simulink model "q2"  (R2020b)
settings: Solver=VariableStepAuto  StartTime=0.0  StopTime=10.0  RelTol=1e-3
values from neighbouring files (symbols this model uses):
  be = 2.0    [clutchpedal_data.sldd]
  bv = 1.0    [clutchpedal_data.sldd]
  Ie = 1.0    [clutchpedal_data.sldd]
  Iv = 5.0    [clutchpedal_data.sldd]
  muk = 1.0    [clutchpedal_data.sldd]
  mus = 1.5    [clutchpedal_data.sldd]
  R = 1.0    [clutchpedal_data.sldd]
settings Model: DataDictionary=clutchpedal_data.sldd  OrderedModelArguments=off  Creator=Ravi  LastModifiedBy=Ravi

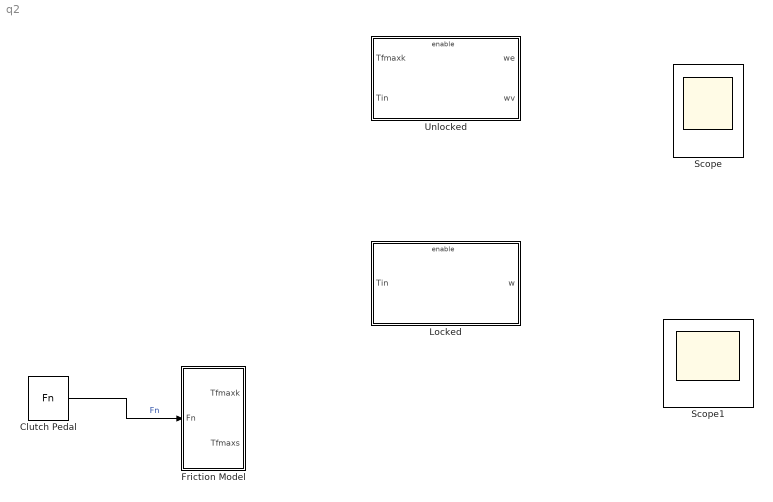
== system q2 ==
  Clutch Pedal : FromWorkspace  VariableName=Fn
  Friction Model : Subsystem
  Locked : Subsystem
  Scope : Scope  NumInputPorts=4
  Scope1 : Scope  NumInputPorts=4
  Unlocked : Subsystem
  wires:
  Clutch Pedal/1 -> Friction Model/1(Fn)  "Fn"

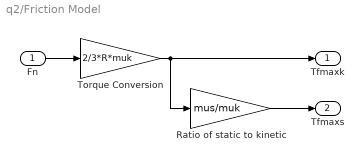
== system q2/Friction Model ==
  Fn : Inport
  Ratio of static to kinetic : Gain  Gain=mus/muk  SaturateOnIntegerOverflow=on  OutDataTypeStr=Inherit: Same as input  ParamDataTypeStr=Inherit: Same as input
  Torque Conversion : Gain  Gain=2/3*R*muk  SaturateOnIntegerOverflow=on  OutDataTypeStr=Inherit: Same as input  ParamDataTypeStr=Inherit: Same as input
  Tfmaxk : Outport  InitialOutput=0  VectorParamsAs1DForOutWhenUnconnected=off
  Tfmaxs : Outport  Port=2  InitialOutput=0  VectorParamsAs1DForOutWhenUnconnected=off
  wires:
  Ratio of static to kinetic/1 -> Tfmaxs/1
  Torque Conversion/1 -> Tfmaxk/1, Ratio of static to kinetic/1
  Fn/1 -> Torque Conversion/1

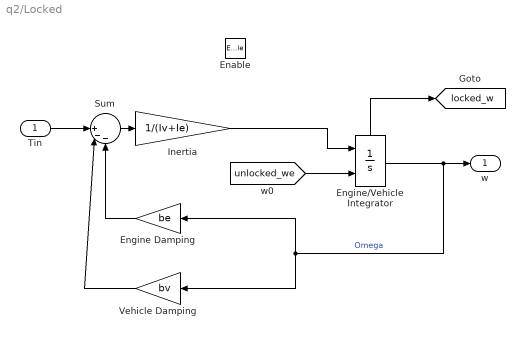
== system q2/Locked ==
  Tin : Inport
  Enable : EnablePort  StatesWhenEnabling=reset
  Engine Damping : Gain  Gain=be  SaturateOnIntegerOverflow=on  OutDataTypeStr=Inherit: Same as input  ParamDataTypeStr=Inherit: Same as input
  Engine/Vehicle Integrator : Integrator  InitialConditionSource=external  ShowStatePort=on
  Inertia : Gain  Gain=1/(Iv+Ie)  SaturateOnIntegerOverflow=on  OutDataTypeStr=Inherit: Same as input  ParamDataTypeStr=Inherit: Same as input
  Sum : Sum  Inputs=||+--  InputSameDT=on  SaturateOnIntegerOverflow=on  OutDataTypeStr=Inherit: Same as first input
  Vehicle Damping : Gain  Gain=bv  SaturateOnIntegerOverflow=on  OutDataTypeStr=Inherit: Same as input  ParamDataTypeStr=Inherit: Same as input
  w : Outport  InitialOutput=0  VectorParamsAs1DForOutWhenUnconnected=off
  tag scope: locked_w=global
  wires:
  Vehicle Damping/1 -> Sum/2
  Inertia/1 -> Engine/Vehicle Integrator/1
  Engine Damping/1 -> Sum/3
  Engine/Vehicle Integrator/1 -> Vehicle Damping/1, Engine Damping/1, w/1  "Omega"
  Tin/1 -> Sum/1
  Sum/1 -> Inertia/1
  Engine/Vehicle Integrator/State -> [locked_w]
  [unlocked_we] -> Engine/Vehicle Integrator/2

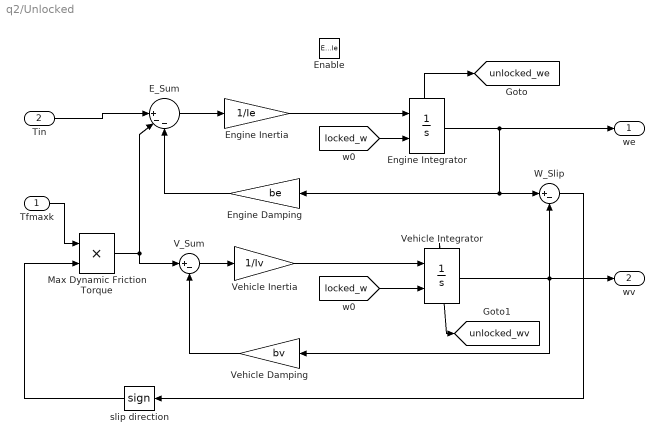
== system q2/Unlocked ==
  Tfmaxk : Inport
  Tin : Inport  Port=2
  Enable : EnablePort  StatesWhenEnabling=reset
  E_Sum : Sum  Inputs=||+--  InputSameDT=on  SaturateOnIntegerOverflow=on  OutDataTypeStr=Inherit: Same as first input
  Engine Damping : Gain  Gain=be  SaturateOnIntegerOverflow=on  OutDataTypeStr=Inherit: Same as input  ParamDataTypeStr=Inherit: Same as input
  Engine Inertia : Gain  Gain=1/Ie  SaturateOnIntegerOverflow=on  OutDataTypeStr=Inherit: Same as input  ParamDataTypeStr=Inherit: Same as input
  Engine Integrator : Integrator  InitialConditionSource=external  ShowStatePort=on
  Max Dynamic Friction Torque : Product  InputSameDT=on  RndMeth=Zero  SaturateOnIntegerOverflow=on  OutDataTypeStr=Inherit: Same as first input
  V_Sum : Sum  Inputs=|+-  InputSameDT=on  SaturateOnIntegerOverflow=on  OutDataTypeStr=Inherit: Same as first input
  Vehicle Integrator : Integrator  InitialConditionSource=external  ShowStatePort=on
  Vehicle Damping : Gain  Gain=bv  SaturateOnIntegerOverflow=on  OutDataTypeStr=Inherit: Same as input  ParamDataTypeStr=Inherit: Same as input
  Vehicle Inertia : Gain  Gain=1/Iv  SaturateOnIntegerOverflow=on  OutDataTypeStr=Inherit: Same as input  ParamDataTypeStr=Inherit: Same as input
  W_Slip : Sum  Inputs=|+-  InputSameDT=on  SaturateOnIntegerOverflow=on  OutDataTypeStr=Inherit: Same as first input
  slip direction : Signum
  we : Outport  InitialOutput=0  VectorParamsAs1DForOutWhenUnconnected=off
  wv : Outport  Port=2  InitialOutput=0  VectorParamsAs1DForOutWhenUnconnected=off
  tag scope: unlocked_we=global, unlocked_wv=global
  wires:
  Engine Integrator/State -> [unlocked_we]
  Vehicle Integrator/1 -> Vehicle Damping/1, wv/1, W_Slip/2
  Tfmaxk/1 -> Max Dynamic Friction Torque/1
  Vehicle Integrator/State -> [unlocked_wv]
  Vehicle Inertia/1 -> Vehicle Integrator/1
  [locked_w] -> Vehicle Integrator/2
  [locked_w] -> Engine Integrator/2
  Tin/1 -> E_Sum/1
  Engine Damping/1 -> E_Sum/3
  slip direction/1 -> Max Dynamic Friction Torque/2
  E_Sum/1 -> Engine Inertia/1
  Engine Inertia/1 -> Engine Integrator/1
  Engine Integrator/1 -> we/1, W_Slip/1, Engine Damping/1
  Max Dynamic Friction Torque/1 -> V_Sum/1, E_Sum/2
  Vehicle Damping/1 -> V_Sum/2
  V_Sum/1 -> Vehicle Inertia/1
  W_Slip/1 -> slip direction/1
